simulink model "GananciaEncoders"  (R2023b)
settings: Solver=VariableStepAuto  StartTime=0.0  StopTime=10.0  RelTol=1e-3
libraries: arduinosensorlib x2, simulink x1
settings Model: Creator=manu_  LastModifiedBy=manu_

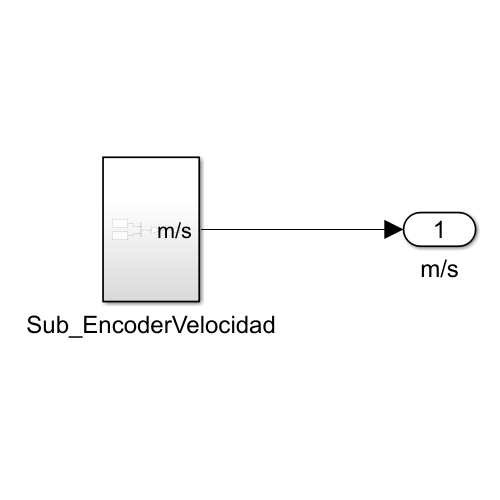
[thumbnail: Simulink's stored preview of the top-level diagram]
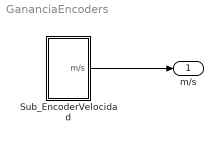
== system GananciaEncoders ==
  Sub_EncoderVelocidad : Subsystem
  m/s : Outport
  wires:
  Sub_EncoderVelocidad/1(m/s) -> m/s/1

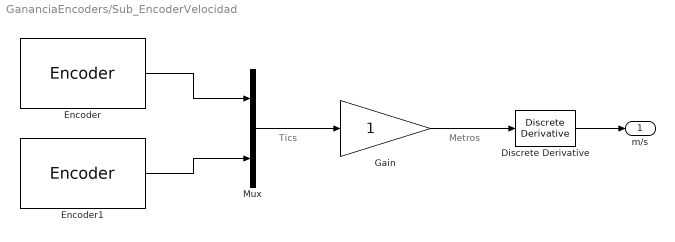
== system GananciaEncoders/Sub_EncoderVelocidad ==
  note: Tics
  note: Metros
  Discrete Derivative : simulink/Discrete/Discrete Derivative  gainval=1.0  ICPrevScaledInput=0.0  OutMin=[]  OutMax=[]  OutDataType=fixdt(1, 16)  OutScaling=2^-10  DoSatur=off
  Encoder : arduinosensorlib/Encoder  InputA=18  InputB=19  Mode=No reset  SampleTime=0.01
  Encoder1 : arduinosensorlib/Encoder  InputA=20  InputB=21  Mode=No reset  SampleTime=0.01
  Gain : Gain
  Mux : Mux  Inputs=2
  m/s : Outport
  wires:
  Encoder1/1 -> Mux/2
  Gain/1 -> Discrete Derivative/1
  Encoder/1 -> Mux/1
  Mux/1 -> Gain/1
  Discrete Derivative/1 -> m/s/1
